simulink model "pg8"  (R2025a)
settings: Solver=VariableStepAuto  StartTime=0.0  StopTime=50  RelTol=1e-3
libraries: dspfdesign x2
settings Model: Creator=Student  LastModifiedBy=Student

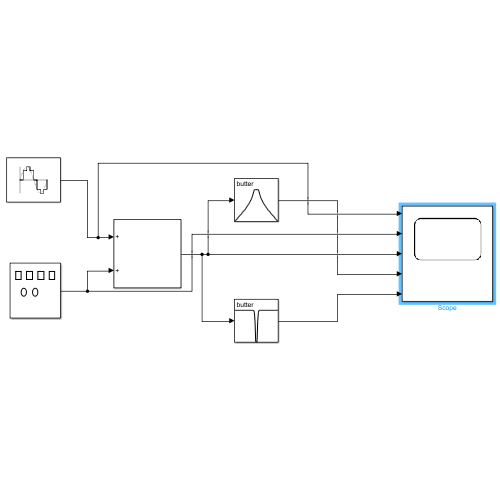
[thumbnail: Simulink's stored preview of the top-level diagram]
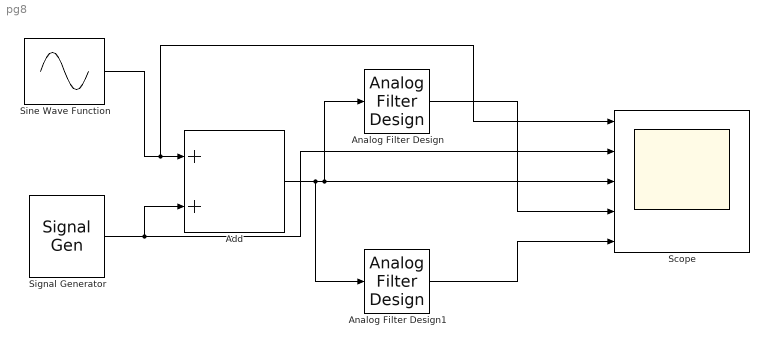
== system pg8 ==
  Add : Sum
  Analog Filter Design : dspfdesign/Analog Filter Design  method=Butterworth  filttype=Bandpass  N=8  Wlo=20  Whi=30  Rp=2  Rs=40
  Analog Filter Design1 : dspfdesign/Analog Filter Design  method=Butterworth  filttype=Bandstop  N=8  Wlo=20  Whi=30  Rp=2  Rs=40
  Scope : Scope  NumInputPorts=5
      settings: ActiveDisplayString=5  Title=Band stop filtered signal  ActiveDisplayYMinimum=-4.10259892645532  ActiveDisplayYMaximum=0.97931639576942753  YLabel=amplitude
  Signal Generator : SignalGenerator  WaveForm=random  Frequency=1000  Units=rad/sec
  Sine Wave Function : Sin  Amplitude=2  Frequency=200  SampleTime=1
  wires:
  Sine Wave Function/1 -> Scope/1, Add/1
  Signal Generator/1 -> Scope/2, Add/2
  Add/1 -> Analog Filter Design1/1, Scope/3, Analog Filter Design/1
  Analog Filter Design/1 -> Scope/4
  Analog Filter Design1/1 -> Scope/5
